simulink model "Simulink_workspace"  (R2015a)
settings: Solver=ode45  StartTime=0.0  StopTime=100  RelTol=1e-3
undefined symbols (not defined in the file or in its folder): National_Instruments, PCI
libraries: sldrtlib x2
settings Model: Creator=noolof  LastModifiedBy=noolof

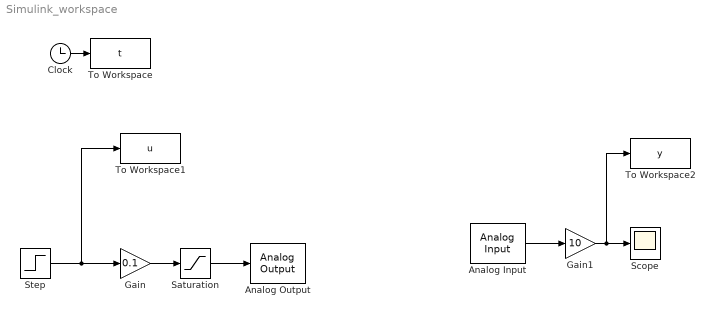
== system Simulink_workspace ==
  Analog Input : sldrtlib/Analog Input  SampleTime=0.01  MaxMissedTicks=100000  ShowMissedTicks=off  YieldWhenWaiting=off  DrvName=National_Instruments/PCI-6014  DrvAddress=4294967295  DrvOptions=[0 0 0 0 0 0]  Channels=1  RangeMode=1  VoltRange=1  DataType=1
      settings: AttributesFormatString=National Instruments\nPCI-6014 [auto]
  Analog Output : sldrtlib/Analog Output  SampleTime=0.01  MaxMissedTicks=1000000  ShowMissedTicks=off  YieldWhenWaiting=off  DrvName=National_Instruments/PCI-6014  DrvAddress=4294967295  DrvOptions=[0 0 0 0 0 0]  Channels=1  RangeMode=1  VoltRange=1  InitialValue=[]  FinalValue=[]
      settings: AttributesFormatString=National Instruments\nPCI-6014 [auto]
  Clock : Clock
  Gain : Gain  Gain=0.1
  Gain1 : Gain  Gain=10
  Saturation : Saturate  UpperLimit=10  LowerLimit=0
  Scope : Scope
      settings: TimeRange=100  YMin=0  YMax=100  SampleInput=on
  Step : Step  Before=48  After=56  SampleTime=0.01
  To Workspace : ToWorkspace  VariableName=t  SampleTime=0.01
  To Workspace1 : ToWorkspace  VariableName=u  SampleTime=0.01
  To Workspace2 : ToWorkspace  VariableName=y  SampleTime=0.01
  wires:
  Step/1 -> To Workspace1/1, Gain/1
  Gain/1 -> Saturation/1
  Saturation/1 -> Analog Output/1
  Clock/1 -> To Workspace/1
  Analog Input/1 -> Gain1/1
  Gain1/1 -> To Workspace2/1, Scope/1
